simulink model "z_one_dive_ac"  (R2014a)
settings: Solver=ode45  StartTime=0.0  StopTime=100  RelTol=1e-3
values from neighbouring files (symbols this model uses):
  Sample_Time = 1    [main.m]
libraries: dspsrcs4 x1
settings Model: Creator=User  LastModifiedBy=User

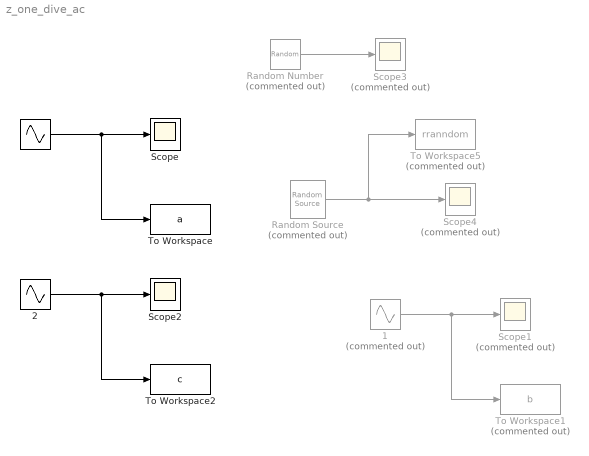
== system z_one_dive_ac ==
  " " : Sin  Amplitude=.489  Bias=.46  Frequency=.03  Phase=-1.1  SampleTime=Sample_Time
  " 1" : Sin  Commented=on  Amplitude=.49/2  Bias=.75  Frequency=.04  Phase=1.57  SampleTime=Sample_Time
  " 2" : Sin  Amplitude=.49  Bias=.5  Frequency=.027  Phase=1.95  SampleTime=Sample_Time
  Random Number : RandomNumber  Commented=on  Mean=0.03  Variance=.0001  Seed=rand  SampleTime=1
  Random Source : dspsrcs4/Random Source  Commented=on  SrcType=Gaussian  NormMethod=Ziggurat  CltLength=12  MinVal=0  MaxVal=1  MeanVal=.1  VarVal=.001  RepMode=Not repeatable  rawSeed=1  IsInherit=on  SampMode=Continuous  SampTime=1  SampFrame=1  DataType=Single  OutComplex=Real
  Scope : Scope
  Scope1 : Scope  Commented=on
  Scope2 : Scope
      settings: SaveName=ScopeData2
  Scope3 : Scope  Commented=on
      settings: SaveName=ScopeData3
  Scope4 : Scope  Commented=on
      settings: SaveName=ScopeData4
  To Workspace : ToWorkspace  VariableName=a  SampleTime=-1
  To Workspace1 : ToWorkspace  Commented=on  VariableName=b  SampleTime=-1
  To Workspace2 : ToWorkspace  VariableName=c  SampleTime=-1
  To Workspace5 : ToWorkspace  Commented=on  VariableName=rranndom  SampleTime=-1
  wires:
  " "/1 -> To Workspace/1, Scope/1
  " 1"/1 -> Scope1/1, To Workspace1/1
  " 2"/1 -> Scope2/1, To Workspace2/1
  Random Number/1 -> Scope3/1
  Random Source/1 -> To Workspace5/1, Scope4/1
